simulink model "pt8612_dpll_fpga_2"  (Simulink 5.0)
settings: Solver=ode45  StartTime=0.0  StopTime=5  RelTol=1e-9  AbsTol=1e-12
values from neighbouring files (symbols this model uses):
  alpha = 2^-24    (= 5.96046447754e-08)    [DPLL_init_2.m]    (also in pt8612_dpll_fpga_init.m = -7; pt8612_dpll_fpga_init_2.m = -5)
  beta = 2^-10    (= 0.0009765625)    [DPLL_init_2.m]    (also in pt8612_dpll_fpga_init.m = 5; pt8612_dpll_fpga_init_2.m = 6)
  C = 680e-9    (= 6.8e-07)    [DPLL_init_2.m]    (also in pt8612_analog_pll_init.m = [1 0]; pt8612_analog_pll_init_2.m = [0 1 0]; pt8612_dpll_fpga_init.m; pt8612_dpll_fpga_init_2.m)
  fvcxo = 148.5e6/1.001    (= 148351648.352)    [DPLL_init_2.m]    (also in pt8612_analog_pll_init.m; pt8612_analog_pll_init_2.m; pt8612_dpll_fpga_init.m; pt8612_dpll_fpga_init_2.m = 148500000)
  Kvcxo = 90e-6    (= 9e-05)    [DPLL_init_2.m]    (also in pt8612_analog_pll_init.m; pt8612_analog_pll_init_2.m; pt8612_dpll_fpga_init.m; pt8612_dpll_fpga_init_2.m)
  Mdac = 3/4    (= 0.75)    [DPLL_init_2.m]    (also in pt8612_dpll_fpga_init.m = 1; pt8612_dpll_fpga_init_2.m = 1)
  Nbits = 16    [DPLL_init_2.m]    (also in pt8612_dpll_fpga_init.m; pt8612_dpll_fpga_init_2.m)
  R = 1/(wkneeloop*20)/C    (= 4060.30501089)    [DPLL_init_2.m]    (also in pt8612_dpll_fpga_init.m; pt8612_dpll_fpga_init_2.m = 3900)
  T = 4*495/fvcxo    (= 1.33333333333e-05)    [pt8612_dpll_fpga_init_2.m]
  time_diff_max = 250/148.5e6    (= 1.6835016835e-06)    [pt8612_dpll_fpga_init_2.m]
  Tlogic = 1/148.5e6    (= 6.73400673401e-09)    [pt8612_dpll_fpga_init_2.m]
  Vcc = 3.3    [DPLL_init_2.m]    (also in pt8612_analog_pll_init.m; pt8612_analog_pll_init_2.m; pt8612_dpll_fpga_init.m = 2.5; pt8612_dpll_fpga_init_2.m = 2.5)
  Vvcxo0 = 1.25    [DPLL_init_2.m]    (also in pt8612_analog_pll_init.m; pt8612_analog_pll_init_2.m; pt8612_dpll_fpga_init.m; pt8612_dpll_fpga_init_2.m)
  Vvcxomax = 2.5    [DPLL_init_2.m]    (also in pt8612_analog_pll_init.m; pt8612_analog_pll_init_2.m; pt8612_dpll_fpga_init.m; pt8612_dpll_fpga_init_2.m)
  Vvcxomin = 0    [DPLL_init_2.m]    (also in pt8612_analog_pll_init.m; pt8612_analog_pll_init_2.m; pt8612_dpll_fpga_init.m; pt8612_dpll_fpga_init_2.m)
libraries: simulink x1
settings Model: LastModifiedBy=thh

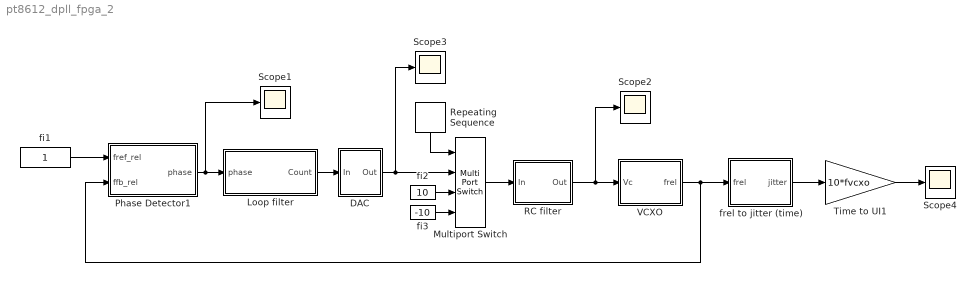
== system pt8612_dpll_fpga_2 ==
  DAC : Subsystem
  Loop filter : Subsystem
  Multiport Switch : MultiPortSwitch  Inputs=3  SaturateOnIntegerOverflow=on
  Phase Detector1 : Subsystem
  RC filter : Subsystem
  Repeating Sequence : simulink/Sources/Repeating Sequence  Orientation=down  rep_seq_t=[0 1 1 2 2 3 3 4]  rep_seq_y=[1 1 2 2 1 1 3 3]
  Scope{1..4} (4 alike) : Scope
      Scope1 settings: TimeRange=10  YMin=-250  YMax=5500  SampleInput=on  SampleTime=T
      Scope2 settings: TimeRange=10  YMin=3.525  YMax=3.9  SaveName=ScopeData3  SampleInput=on  SampleTime=T
      Scope3 settings: TimeRange=10  YMin=0  YMax=2.5  SampleInput=on  SampleTime=T
      Scope4 settings: TimeRange=10  YMin=-3020  YMax=-2977.5  SaveName=ScopeData2  SampleInput=on  SampleTime=1e-4
  Time to UI1 : Gain  Gain=10*fvcxo  SaturateOnIntegerOverflow=on
  VCXO : Subsystem
  fi1 : Constant
  fi2 : Constant  Value=10
  fi3 : Constant  Value=-10
  frel to jitter (time) : Subsystem
  wires:
  frel to jitter (time)/1(jitter) -> Time to UI1/1
  Time to UI1/1 -> Scope4/1
  Phase Detector1/1(phase) -> Loop filter/1(phase), Scope1/1
  fi1/1 -> Phase Detector1/1(fref_rel)
  DAC/1(Out) -> Scope3/1, Multiport Switch/2
  VCXO/1(frel) -> frel to jitter (time)/1(frel), Phase Detector1/2(ffb_rel)
  Loop filter/1(Count) -> DAC/1(In)
  Multiport Switch/1 -> RC filter/1(In)
  fi2/1 -> Multiport Switch/3
  fi3/1 -> Multiport Switch/4
  Repeating Sequence/1 -> Multiport Switch/1
  RC filter/1(Out) -> VCXO/1(Vc), Scope2/1

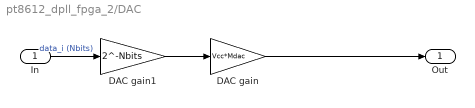
== system pt8612_dpll_fpga_2/DAC ==
  In : Inport
  DAC gain : Gain  Gain=Vcc*Mdac  SaturateOnIntegerOverflow=on
  DAC gain1 : Gain  Gain=2^-Nbits  SaturateOnIntegerOverflow=on
  Out : Outport
  wires:
  In/1 -> DAC gain1/1  "data_i (Nbits)"
  DAC gain/1 -> Out/1
  DAC gain1/1 -> DAC gain/1

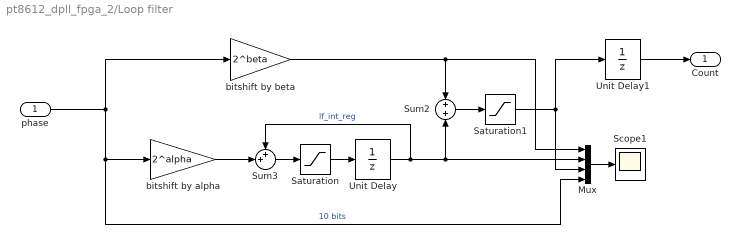
== system pt8612_dpll_fpga_2/Loop filter ==
  phase : Inport
  Mux : Mux
  Saturation : Saturate  UpperLimit=2^16  LowerLimit=0
  Saturation1 : Saturate  UpperLimit=2^16  LowerLimit=0
  Scope1 : Scope
      settings: TimeRange=10  YMin=-20000  YMax=70000  SaveName=ScopeData5  Decimation=100  SampleTime=T
  Sum2 : Sum  SaturateOnIntegerOverflow=on
  Sum3 : Sum  Inputs=++|  SaturateOnIntegerOverflow=on
  Unit Delay : UnitDelay  SampleTime=T
  Unit Delay1 : UnitDelay  SampleTime=T
  bitshift by alpha : Gain  Gain=2^alpha  SaturateOnIntegerOverflow=on
  bitshift by beta : Gain  Gain=2^beta  SaturateOnIntegerOverflow=on
  Count : Outport
  wires:
  phase/1 -> bitshift by beta/1, Mux/4, bitshift by alpha/1  "10 bits"
  Sum2/1 -> Saturation1/1
  bitshift by beta/1 -> Sum2/1, Mux/1
  Mux/1 -> Scope1/1
  Unit Delay/1 -> Sum2/2, Mux/2, Sum3/1  "lf_int_reg"
  Sum3/1 -> Saturation/1
  Unit Delay1/1 -> Count/1
  bitshift by alpha/1 -> Sum3/2
  Saturation/1 -> Unit Delay/1
  Saturation1/1 -> Mux/3, Unit Delay1/1

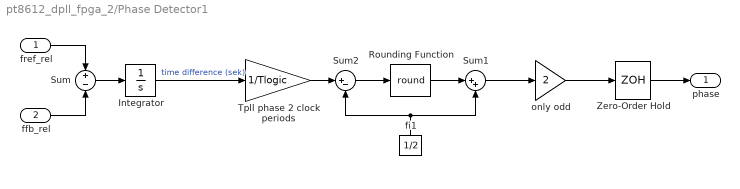
== system pt8612_dpll_fpga_2/Phase Detector1 ==
  fref_rel : Inport
  ffb_rel : Inport  Port=2
  Integrator : Integrator  LimitOutput=on  UpperSaturationLimit=time_diff_max  LowerSaturationLimit=-time_diff_max
  Rounding Function : Rounding  Operator=round
  Sum : Sum  Inputs=+-  SaturateOnIntegerOverflow=on
  Sum1 : Sum  Inputs=|++  SaturateOnIntegerOverflow=on
  Sum2 : Sum  Inputs=|+-  SaturateOnIntegerOverflow=on
  Tpll phase 2 clock periods : Gain  Gain=1/Tlogic  SaturateOnIntegerOverflow=on
  Zero-Order Hold : ZeroOrderHold  SampleTime=T
  fi1 : Constant  Orientation=up  Value=1/2
  only odd : Gain  Gain=2  SaturateOnIntegerOverflow=on
  phase : Outport
  wires:
  ffb_rel/1 -> Sum/2
  fref_rel/1 -> Sum/1
  Sum/1 -> Integrator/1
  Integrator/1 -> Tpll phase 2 clock periods/1  "time difference (sek)"
  fi1/1 -> Sum1/2, Sum2/2
  Sum2/1 -> Rounding Function/1
  Sum1/1 -> only odd/1
  Rounding Function/1 -> Sum1/1
  Tpll phase 2 clock periods/1 -> Sum2/1
  Zero-Order Hold/1 -> phase/1
  only odd/1 -> Zero-Order Hold/1

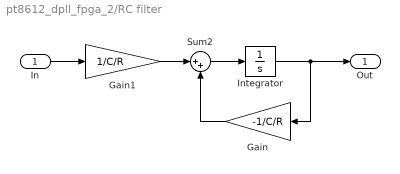
== system pt8612_dpll_fpga_2/RC filter ==
  In : Inport
  Gain : Gain  Orientation=left  Gain=-1/C/R  SaturateOnIntegerOverflow=on
  Gain1 : Gain  Gain=1/C/R  SaturateOnIntegerOverflow=on
  Integrator : Integrator  InitialCondition=Vvcxo0
  Sum2 : Sum  Inputs=|++  SaturateOnIntegerOverflow=on
  Out : Outport
  wires:
  In/1 -> Gain1/1
  Integrator/1 -> Out/1, Gain/1
  Sum2/1 -> Integrator/1
  Gain/1 -> Sum2/2
  Gain1/1 -> Sum2/1

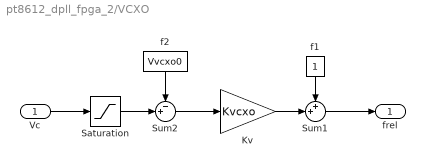
== system pt8612_dpll_fpga_2/VCXO ==
  Vc : Inport
  Kv : Gain  Gain=Kvcxo  SaturateOnIntegerOverflow=on
  Saturation : Saturate  UpperLimit=Vvcxomax  LowerLimit=Vvcxomin
  Sum1 : Sum  Inputs=++|  SaturateOnIntegerOverflow=on
  Sum2 : Sum  Inputs=-+|  SaturateOnIntegerOverflow=on
  f1 : Constant  Orientation=down
  f2 : Constant  Orientation=down  Value=Vvcxo0
  frel : Outport
  wires:
  f2/1 -> Sum2/1
  Vc/1 -> Saturation/1
  Sum2/1 -> Kv/1
  Kv/1 -> Sum1/2
  f1/1 -> Sum1/1
  Saturation/1 -> Sum2/2
  Sum1/1 -> frel/1

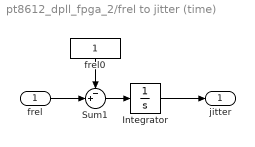
== system pt8612_dpll_fpga_2/frel to jitter (time) ==
  frel : Inport
  Integrator : Integrator
  Sum1 : Sum  Inputs=-+|  SaturateOnIntegerOverflow=on
  frel0 : Constant  Orientation=down
  jitter : Outport
  wires:
  frel/1 -> Sum1/2
  frel0/1 -> Sum1/1
  Sum1/1 -> Integrator/1
  Integrator/1 -> jitter/1
